simulink model "liti4_7xiti1"  (Simulink 5.0)
settings: Solver=ode4  SolverMode=SingleTasking  StartTime=0.0  StopTime=8  FixedStep=0.001  RelTol=1e-3
settings Model: LastModifiedBy=Administrator

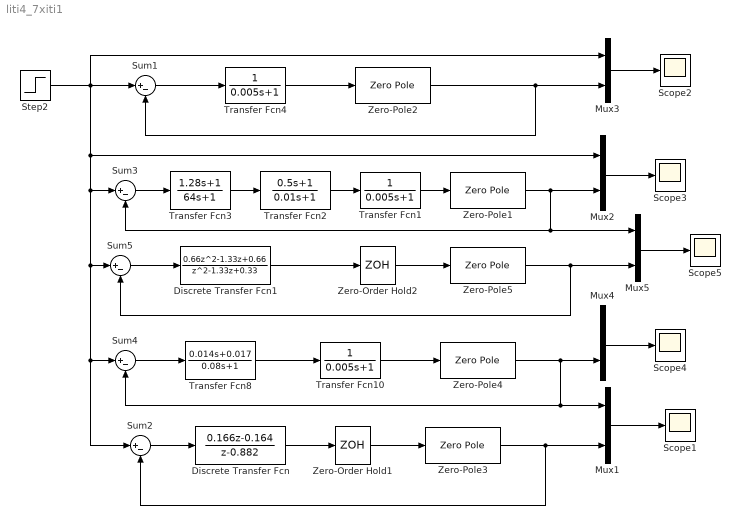
== system liti4_7xiti1 ==
  Discrete Transfer Fcn : DiscreteTransferFcn  Numerator=[0.166 -0.164]  Denominator=[1 -0.882]  SampleTime=0.01
  Discrete Transfer Fcn1 : DiscreteTransferFcn  Numerator=[0.66 -1.33 0.66]  Denominator=[1 -1.33 0.33]  SampleTime=0.01
  Mux{1..5} (5 alike) : Mux  Inputs=2
  Scope{1..5} (5 alike) : Scope
      Scope1 settings: YMin=-3.5  YMax=1  SaveName=yyy  DataFormat=Array  MaxDataPoints=500000
      Scope2 settings: YMin=-3.5  YMax=1  MaxDataPoints=500000
      Scope3 settings: YMin=-3.5  YMax=1  SaveName=ScopeData2  MaxDataPoints=500000
      Scope4 settings: YMin=-3.5  YMax=1  SaveName=ScopeData3  MaxDataPoints=500000
      Scope5 settings: YMin=-3.5  YMax=1  SaveName=yyy1  DataFormat=Array  MaxDataPoints=500000
  Step2 : Step  Time=0  SampleTime=0
  Sum{1..5} (5 alike) : Sum  Inputs=|+-  SaturateOnIntegerOverflow=on
  Transfer Fcn1 : TransferFcn  Denominator=[0.005 1]
  Transfer Fcn10 : TransferFcn  Denominator=[0.005 1]
  Transfer Fcn2 : TransferFcn  Numerator=[0.5 1]  Denominator=[0.01 1]
  Transfer Fcn3 : TransferFcn  Numerator=[1.28 1]  Denominator=[64 1]
  Transfer Fcn4 : TransferFcn  Denominator=[0.005 1]
  Transfer Fcn8 : TransferFcn  Numerator=[0.014 0.017]  Denominator=[0.08 1]
  Zero-Order Hold1 : ZeroOrderHold  SampleTime=0.01
  Zero-Order Hold2 : ZeroOrderHold  SampleTime=0.01
  Zero-Pole{1..5} (5 alike) : ZeroPole  Zeros=[]  Poles=[0 -6 -2]  Gain=[12*180]
  wires:
  Step2/1 -> Sum3/1, Sum4/1, Sum2/1, Sum5/1, Mux2/1, Mux3/1, Sum1/1
  Mux2/1 -> Scope3/1
  Zero-Pole1/1 -> Mux2/2, Sum3/2, Mux5/1
  Mux3/1 -> Scope2/1
  Zero-Pole2/1 -> Mux3/2, Sum1/2
  Sum1/1 -> Transfer Fcn4/1
  Sum3/1 -> Transfer Fcn3/1
  Transfer Fcn3/1 -> Transfer Fcn2/1
  Transfer Fcn4/1 -> Zero-Pole2/1
  Transfer Fcn2/1 -> Transfer Fcn1/1
  Mux4/1 -> Scope4/1
  Zero-Pole4/1 -> Mux4/2, Sum4/2, Mux1/1
  Sum4/1 -> Transfer Fcn8/1
  Transfer Fcn8/1 -> Transfer Fcn10/1
  Transfer Fcn10/1 -> Zero-Pole4/1
  Mux1/1 -> Scope1/1
  Zero-Pole3/1 -> Mux1/2, Sum2/2
  Discrete Transfer Fcn/1 -> Zero-Order Hold1/1
  Sum2/1 -> Discrete Transfer Fcn/1
  Zero-Order Hold1/1 -> Zero-Pole3/1
  Transfer Fcn1/1 -> Zero-Pole1/1
  Mux5/1 -> Scope5/1
  Zero-Pole5/1 -> Sum5/2, Mux5/2
  Discrete Transfer Fcn1/1 -> Zero-Order Hold2/1
  Sum5/1 -> Discrete Transfer Fcn1/1
  Zero-Order Hold2/1 -> Zero-Pole5/1
